simulink model "A_Justo_SCHFV_slx_UFHDV_Design_NoLinGS"  (R2019a)
settings: Solver=VariableStepAuto  StartTime=0.0  StopTime=tfinal  MaxStep=maxstepsize  RelTol=1e-3  EnableMultiTasking=on
values from neighbouring files (symbols this model uses):
  aini = 0    [A_Justo_SCHFV_m_UFHDV_Design.m]
  eta = sum(normrnd(IDM_t,IDM_ts,1,n))    [A_Justo_SCHFV_m_Control_Sensitivity.m]    (also in A_Justo_SCHFV_m_UFHDV_Design.m; TransferFunctionPROP.m = IDM_T(acc1+n1,acc1+n1))
  hini = 1.01*IDM_H0    [A_Justo_SCHFV_m_UFHDV_Design.m]
  IDM_Amax = IDM_Amax(acc1+n1,acc1+n1)    [TransferFunctionPROP.m]
  IDM_Bmax = IDM_Bmax(acc1+n1,acc1+n1)    [TransferFunctionPROP.m]
  IDM_Delta = IDM_Delta(acc1+n1)    [TransferFunctionPROP.m]
  IDM_H0 = IDM_H0(acc1+n1)    [TransferFunctionPROP.m]
  IDM_T = normrnd(IDM_t,IDM_ts)    [A_Justo_SCHFV_m_Control_Sensitivity.m]    (also in A_Justo_SCHFV_m_Track.m = IDM_Tind; A_Justo_SCHFV_m_UFHDV_Design.m; TransferFunctionPROP.m = IDM_T(acc1+n1,acc1+n1))
  IDM_V0 = IDM_V0(acc1+n1)    [TransferFunctionPROP.m]
  kgain = 0.02    [A_Justo_SCHFV_m_Track.m]    (also in A_Justo_SCHFV_m_UFHDV_Design.m)
  Lini = Lind    [A_Justo_SCHFV_m_Track.m]    (also in A_Justo_SCHFV_m_UFHDV_Design.m = sum(normrnd(l,ls,1,n)))
  P = [pDom; conj(pDom); pNeg1; pNeg2; pNeg3; pNeg4]    [A_Justo_SCHFV_m_Control_Sensitivity.m]    (also in A_Justo_SCHFV_m_UFHDV_Design.m)
  Tau_A = normrnd(tau,taus)    [A_Justo_SCHFV_m_Control_Sensitivity.m]    (also in A_Justo_SCHFV_m_UFHDV_Design.m; TransferFunctionPROP.m = Tau(acc1,acc1))
  Tau_H = normrnd(tau,taus)    [A_Justo_SCHFV_m_Control_Sensitivity.m]    (also in A_Justo_SCHFV_m_UFHDV_Design.m; TransferFunctionPROP.m = Tau(acc1+n1,acc1+n1))
  v_r_0 = 30/3.6    (= 8.33333333333)    [A_Justo_SCHFV_m_Control_Sensitivity.m]    (also in A_Justo_SCHFV_m_Track.m = 5.55555555556; A_Justo_SCHFV_m_UFHDV_Design.m = 2.77777777778)
  vini = 0    [A_Justo_SCHFV_m_UFHDV_Design.m]
  zini = 0    [A_Justo_SCHFV_m_UFHDV_Design.m]
settings Model: Creator=arnaudoria  LastModifiedBy=Sander
settings DataIOCC: LimitDataPoints=on  ReturnWorkspaceOutputs=off
settings OptimizationCC: LifeSpan=inf
settings DebuggingCC: AllowSymbolicDim=off  SFUnexpectedBacktrackingDiag=warning  SFNoUnconditionalDefaultTransitionDiag=warning  SFExecutionAtInitializationDiag=none  ArithmeticOperatorsInVariantConditions=warning
settings ModelReferenceCC: PropagateSignalLabelsOutOfModel=off
settings SFSimCC: SimUseLocalCustomCode=off
settings RTWCC: RTWUseLocalCustomCode=off
settings CodeAppCC: StateflowObjectComments=on
settings GRTTargetCC: TargetLangStandard=C89/C90 (ANSI)
settings ConfigComp: CovMetricSettings=dw  CovHtmlReporting=on  CovSaveCumulativeToWorkspaceVar=on  CovSaveSingleToWorkspaceVar=on  CovExternalEMLEnable=off

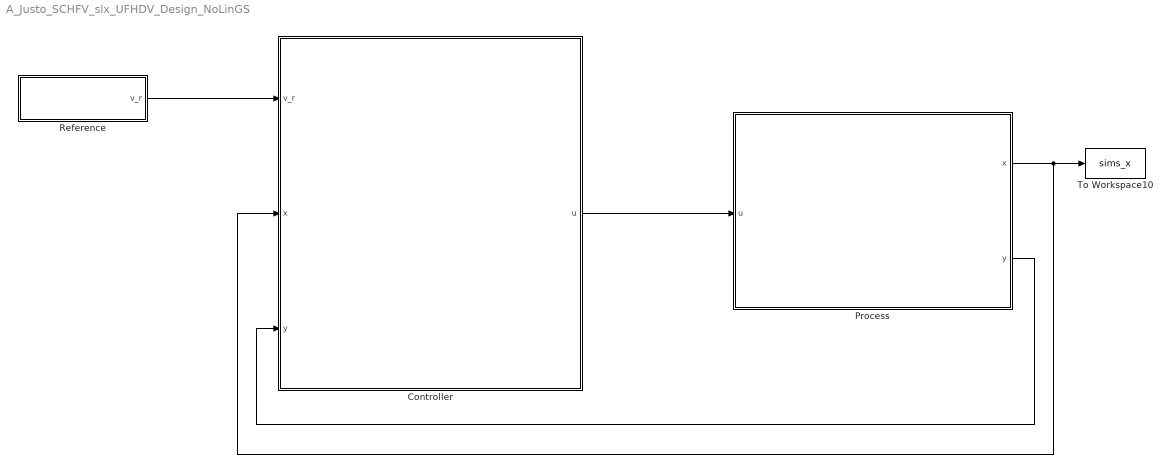
== system A_Justo_SCHFV_slx_UFHDV_Design_NoLinGS ==
  Controller : Subsystem
  Process : Subsystem
  Reference : Subsystem
  To Workspace10 : ToWorkspace  VariableName=sims_x  SampleTime=-1
  wires:
  Controller/1(u) -> Process/1(u)
  Process/2(y) -> Controller/3(y)
  Process/1(x) -> Controller/2(x), To Workspace10/1
  Reference/1(v_r) -> Controller/1(v_r)

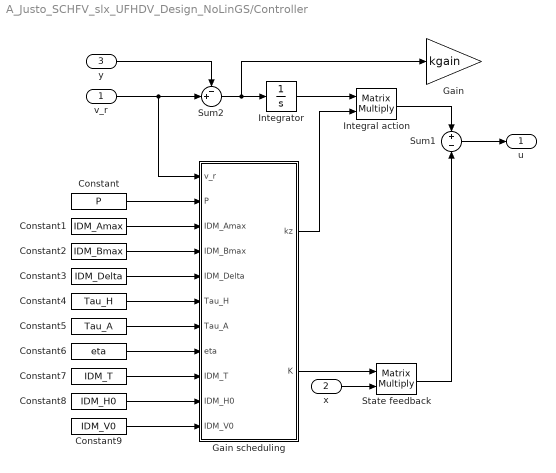
== system A_Justo_SCHFV_slx_UFHDV_Design_NoLinGS/Controller ==
  v_r : Inport
  x : Inport  Port=2
  y : Inport  Port=3
  Constant : Constant  Value=P
  Constant1 : Constant  Value=IDM_Amax
  Constant2 : Constant  Value=IDM_Bmax
  Constant3 : Constant  Value=IDM_Delta
  Constant4 : Constant  Value=Tau_H
  Constant5 : Constant  Value=Tau_A
  Constant6 : Constant  Value=eta
  Constant7 : Constant  Value=IDM_T
  Constant8 : Constant  Value=IDM_H0
  Constant9 : Constant  Value=IDM_V0
  Gain : Gain  Gain=kgain
  Gain scheduling : MATLAB Function  TreatAsAtomicUnit=on
  Integral action : Product  Multiplication=Matrix(*)
  Integrator : Integrator  InitialCondition=zini
  State feedback : Product  Multiplication=Matrix(*)
  Sum1 : Sum  Inputs=+|-
  Sum2 : Sum  Inputs=-+|
  u : Outport
  wires:
  Integrator/1 -> Integral action/1
  Integral action/1 -> Sum1/1
  x/1 -> State feedback/2
  Constant/1 -> Gain scheduling/2(P)
  Constant1/1 -> Gain scheduling/3(IDM_Amax)
  Constant2/1 -> Gain scheduling/4(IDM_Bmax)
  Constant3/1 -> Gain scheduling/5(IDM_Delta)
  Constant4/1 -> Gain scheduling/6(Tau_H)
  Constant5/1 -> Gain scheduling/7(Tau_A)
  Constant6/1 -> Gain scheduling/8(eta)
  Constant7/1 -> Gain scheduling/9(IDM_T)
  Constant8/1 -> Gain scheduling/10(IDM_H0)
  Constant9/1 -> Gain scheduling/11(IDM_V0)
  State feedback/1 -> Sum1/2
  Gain scheduling/2(K) -> State feedback/1
  Gain scheduling/1(kz) -> Integral action/2
  y/1 -> Sum2/1
  v_r/1 -> Sum2/2, Gain scheduling/1(v_r)
  Sum2/1 -> Integrator/1, Gain/1
  Sum1/1 -> u/1

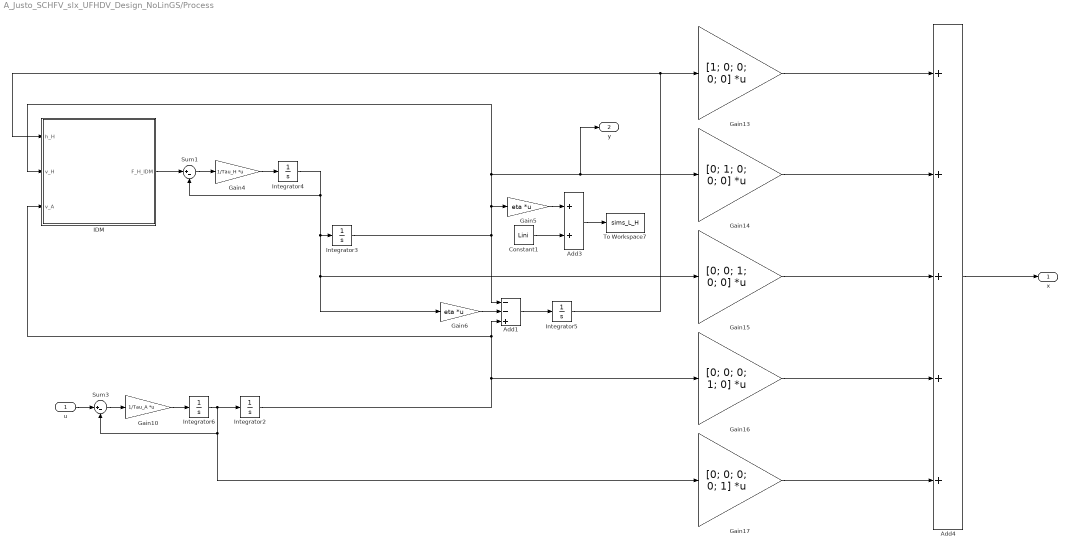
== system A_Justo_SCHFV_slx_UFHDV_Design_NoLinGS/Process ==
  u : Inport
  Add1 : Sum  Inputs=--+
  Add3 : Sum
  Add4 : Sum  Inputs=+++++
  Constant1 : Constant  Value=Lini
  Gain10 : Gain  Gain=1/Tau_A  Multiplication=Matrix(K*u)
  Gain13 : Gain  Gain=[1; 0; 0; 0; 0]  Multiplication=Matrix(K*u)
  Gain14 : Gain  Gain=[0; 1; 0; 0; 0]  Multiplication=Matrix(K*u)
  Gain15 : Gain  Gain=[0; 0; 1; 0; 0]  Multiplication=Matrix(K*u)
  Gain16 : Gain  Gain=[0; 0; 0; 1; 0]  Multiplication=Matrix(K*u)
  Gain17 : Gain  Gain=[0; 0; 0; 0; 1]  Multiplication=Matrix(K*u)
  Gain4 : Gain  Gain=1/Tau_H  Multiplication=Matrix(K*u)
  Gain5 : Gain  Gain=eta  Multiplication=Matrix(K*u)
  Gain6 : Gain  Gain=eta  Multiplication=Matrix(K*u)
  IDM : Subsystem
  Integrator2 : Integrator  InitialCondition=vini  WrappedStateUpperValue=2*pi  WrappedStateLowerValue=0
  Integrator3 : Integrator  InitialCondition=vini  WrappedStateUpperValue=2*pi  WrappedStateLowerValue=0
  Integrator4 : Integrator  InitialCondition=aini  WrappedStateUpperValue=2*pi  WrappedStateLowerValue=0
  Integrator5 : Integrator  InitialCondition=hini  WrappedStateUpperValue=2*pi  WrappedStateLowerValue=0
  Integrator6 : Integrator  InitialCondition=aini  WrappedStateUpperValue=2*pi  WrappedStateLowerValue=0
  Sum1 : Sum  Inputs=|+-
  Sum3 : Sum  Inputs=|+-
  To Workspace7 : ToWorkspace  VariableName=sims_L_H  SampleTime=-1
  x : Outport
  y : Outport  Port=2
  wires:
  u/1 -> Sum3/1
  Add1/1 -> Integrator5/1
  Gain5/1 -> Add3/1
  Integrator6/1 -> Gain17/1, Sum3/2, Integrator2/1
  Integrator4/1 -> Integrator3/1, Gain6/1, Gain15/1, Sum1/2
  Constant1/1 -> Add3/2
  Add3/1 -> To Workspace7/1
  Sum3/1 -> Gain10/1
  Gain10/1 -> Integrator6/1
  Integrator5/1 -> IDM/1(h_H), Gain13/1
  Sum1/1 -> Gain4/1
  Gain4/1 -> Integrator4/1
  Integrator3/1 -> Add1/1, IDM/2(v_H), Gain14/1, y/1, Gain5/1
  Gain17/1 -> Add4/5
  Gain16/1 -> Add4/4
  Gain15/1 -> Add4/3
  Gain14/1 -> Add4/2
  Gain13/1 -> Add4/1
  Add4/1 -> x/1
  Gain6/1 -> Add1/2
  IDM/1(F_H_IDM) -> Sum1/1
  Integrator2/1 -> Add1/3, IDM/3(v_A), Gain16/1

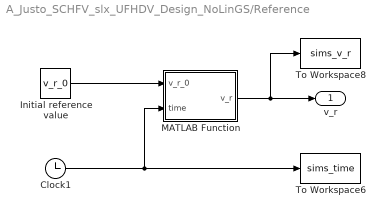
== system A_Justo_SCHFV_slx_UFHDV_Design_NoLinGS/Reference ==
  Clock1 : Clock
  Initial reference value : Constant  Value=v_r_0
  MATLAB Function : MATLAB Function  TreatAsAtomicUnit=on
  To Workspace6 : ToWorkspace  VariableName=sims_time  SampleTime=-1
  To Workspace8 : ToWorkspace  VariableName=sims_v_r  SampleTime=-1
  v_r : Outport
  wires:
  Clock1/1 -> To Workspace6/1, MATLAB Function/2(time)
  MATLAB Function/1(v_r) -> v_r/1, To Workspace8/1
  Initial reference value/1 -> MATLAB Function/1(v_r_0)

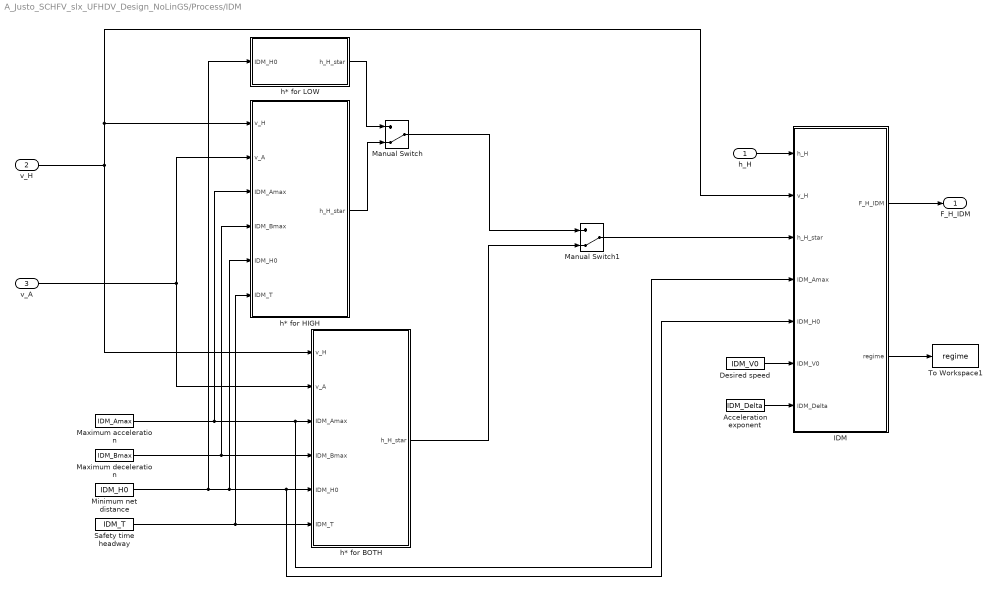
== system A_Justo_SCHFV_slx_UFHDV_Design_NoLinGS/Process/IDM ==
  h_H : Inport
  v_H : Inport  Port=2
  v_A : Inport  Port=3
  Acceleration exponent : Constant  Value=IDM_Delta
  Desired speed : Constant  Value=IDM_V0
  IDM : MATLAB Function  TreatAsAtomicUnit=on
  Manual Switch : ManualSwitch  CurrentSetting=0
  Manual Switch1 : ManualSwitch  CurrentSetting=0
  Maximum acceleration : Constant  Value=IDM_Amax
  Maximum deceleration : Constant  Value=IDM_Bmax
  Minimum net distance : Constant  Value=IDM_H0
  Safety time headway : Constant  Value=IDM_T
  To Workspace1 : ToWorkspace  VariableName=regime  SampleTime=-1
  h* for BOTH : MATLAB Function  TreatAsAtomicUnit=on
  h* for HIGH : MATLAB Function  TreatAsAtomicUnit=on
  h* for LOW : MATLAB Function  TreatAsAtomicUnit=on
  F_H_IDM : Outport
  wires:
  Acceleration exponent/1 -> IDM/7(IDM_Delta)
  Desired speed/1 -> IDM/6(IDM_V0)
  IDM/2(regime) -> To Workspace1/1
  IDM/1(F_H_IDM) -> F_H_IDM/1
  Minimum net distance/1 -> h* for HIGH/5(IDM_H0), h* for BOTH/5(IDM_H0), IDM/5(IDM_H0), h* for LOW/1(IDM_H0)
  Maximum acceleration/1 -> h* for HIGH/3(IDM_Amax), h* for BOTH/3(IDM_Amax), IDM/4(IDM_Amax)
  Safety time headway/1 -> h* for HIGH/6(IDM_T), h* for BOTH/6(IDM_T)
  Maximum deceleration/1 -> h* for HIGH/4(IDM_Bmax), h* for BOTH/4(IDM_Bmax)
  h_H/1 -> IDM/1(h_H)
  h* for LOW/1(h_H_star) -> Manual Switch/1
  h* for HIGH/1(h_H_star) -> Manual Switch/2
  Manual Switch/1 -> Manual Switch1/1
  h* for BOTH/1(h_H_star) -> Manual Switch1/2
  Manual Switch1/1 -> IDM/3(h_H_star)
  v_H/1 -> h* for HIGH/1(v_H), IDM/2(v_H), h* for BOTH/1(v_H)
  v_A/1 -> h* for HIGH/2(v_A), h* for BOTH/2(v_A)

== matlab function A_Justo_SCHFV_slx_UFHDV_Design_NoLinGS/Reference/MATLAB Function ==
  data: v_r_0 input; v_r output; time input
function v_r = fcn(v_r_0, time)
v_r = v_r_0;
if time < 100
    v_r = 1*v_r_0;
elseif time >=100 && time <200
    v_r = 2*v_r_0;
elseif time >=200 && time <300
    v_r = 3*v_r_0;
elseif time >=300 && time <500
    v_r = 4*v_r_0;
elseif time >=500 && time <600
    v_r = 3*v_r_0;
elseif time >=600 && time <700
    v_r = 2*v_r_0;
elseif time >=700 && time <800
    v_r = 1*v_r_0;
end
end

== matlab function A_Justo_SCHFV_slx_UFHDV_Design_NoLinGS/Process/IDM/h* for HIGH ==
  data: v_H input; h_H_star output; v_A input; IDM_Amax input; IDM_Bmax input; IDM_H0 input; IDM_T input
function h_H_star = fcn(v_H,v_A,IDM_Amax,IDM_Bmax,IDM_H0,IDM_T)
h_H_star = IDM_H0 + IDM_T*v_H + v_H*(v_H-v_A)/(2*sqrt(IDM_Amax*IDM_Bmax));
end

== matlab function A_Justo_SCHFV_slx_UFHDV_Design_NoLinGS/Process/IDM/h* for LOW ==
  data: h_H_star output; IDM_H0 input
function h_H_star = fcn(IDM_H0)
h_H_star = IDM_H0;
end

== matlab function A_Justo_SCHFV_slx_UFHDV_Design_NoLinGS/Process/IDM/h* for BOTH ==
  data: v_H input; h_H_star output; v_A input; IDM_Amax input; IDM_Bmax input; IDM_H0 input; IDM_T input
function h_H_star = fcn(v_H,v_A,IDM_Amax,IDM_Bmax,IDM_H0,IDM_T)
h_H_star = IDM_H0 + ...
    max( 0, IDM_T*v_H + v_H*(v_H-v_A)/(2*sqrt(IDM_Amax*IDM_Bmax)) );
end

== matlab function A_Justo_SCHFV_slx_UFHDV_Design_NoLinGS/Controller/Gain scheduling ==
  data: kz output; v_r input; K output; P input; IDM_Amax input; IDM_Bmax input; IDM_Delta input; Tau_H input; Tau_A input; eta input; IDM_T input; IDM_H0 input; IDM_V0 input
function [kz,K] = fcn(v_r,P,IDM_Amax,IDM_Bmax,IDM_Delta,Tau_H,Tau_A,eta,IDM_T,IDM_H0,IDM_V0)
kz=0; K=zeros(1,5);
% % Linearized system
% A31 = 2*IDM_Amax/Tau_H/(IDM_H0+v_r*IDM_T)*(1-(v_r/IDM_V0)^IDM_Delta)^(3/2);
% A32 = -IDM_Amax/Tau_H*(IDM_Delta*v_r^(IDM_Delta-1)/IDM_V0^IDM_Delta+(v_r+2*IDM_T*sqrt(IDM_Amax*IDM_Bmax))/((IDM_H0+v_r*IDM_T)*sqrt(IDM_Amax*IDM_Bmax))*(1-(v_r/IDM_V0)^IDM_Delta));
% A34 = IDM_Amax/Tau_H*v_r/((IDM_H0+v_r*IDM_T)*sqrt(IDM_Amax*IDM_Bmax))*(1-(v_r/IDM_V0)^IDM_Delta);
% A = [ 0    -1     -eta      1       0    0 ;...
%       0     0       1       0       0    0 ;...
%      A31   A32  -1/Tau_H   A34      0    0 ;...
%       0     0       0       0       1    0 ;...
%       0     0       0       0   -1/Tau_A 0 ;...
%       0     1       0       0       0    0 ];
% B = [0; 0; 0; 0; 1/Tau_A; 0];
% % Controllability matrix
% W_C = [B A*B A^2*B A^3*B A^4*B A^5*B];
% % Desired polynomial
% P_d = (A-P(1)*eye(6))*(A-P(2)*eye(6))*(A-P(3)*eye(6))*(A-P(4)*eye(6))...
%     *(A-P(5)*eye(6))*(A-P(6)*eye(6));
% % Ackermann's formula
% Kack = [0 0 0 0 0 1]*(W_C\P_d);
% Kack = real(Kack);
% % Gains
% kz = Kack(6); K = [Kack(1) Kack(2) Kack(3) Kack(4) Kack(5)];
% end

== matlab function A_Justo_SCHFV_slx_UFHDV_Design_NoLinGS/Process/IDM/IDM ==
  data: h_H input; v_H input; h_H_star input; IDM_Amax input; IDM_H0 input; IDM_V0 input; IDM_Delta input; F_H_IDM output; regime output
function [F_H_IDM,regime] = fcn(h_H,v_H,h_H_star,IDM_Amax,IDM_H0,IDM_V0,IDM_Delta)
if h_H_star == IDM_H0
    regime=0;
else
    regime=1;
end
%v_H=v_H*(v_H>=0); % RECORDAR QUE SE HA AÑADIDO ESTA SATURACIÓN
F_H_IDM = IDM_Amax*(1-(v_H/IDM_V0)^IDM_Delta-(h_H_star/h_H)^2);
end
